simulink model "abl_M4_rigidPPC"  (R2023b)
settings: Solver=ode45  StartTime=0.0  StopTime=80  MaxStep=1e-3  RelTol=5e-5
model workspace (MAT data in the model file):
  gpsid1 = Simulink.Signal
  gpsid1.DataType = 'double'
  gpsid1.Dimensions = 1
  gpsid1.DimensionsMode = 'auto'
  gpsid1.Complexity = 'real'
  gpsid1.SampleTime = -1
  gpsid1.SamplingMode = 'auto'
  gpsid2 = Simulink.Signal
  gpsid2.DataType = 'double'
  gpsid2.Dimensions = 1
  gpsid2.DimensionsMode = 'auto'
  gpsid2.Complexity = 'real'
  gpsid2.SampleTime = -1
  gpsid2.SamplingMode = 'auto'
  gpsid3 = Simulink.Signal
  gpsid3.DataType = 'double'
  gpsid3.Dimensions = 1
  gpsid3.DimensionsMode = 'auto'
  gpsid3.Complexity = 'real'
  gpsid3.SampleTime = -1
  gpsid3.SamplingMode = 'auto'
  kkk1 = Simulink.Signal
  kkk1.DataType = 'double'
  kkk1.Dimensions = 1
  kkk1.DimensionsMode = 'auto'
  kkk1.Complexity = 'real'
  kkk1.SampleTime = -1
  kkk1.SamplingMode = 'auto'
  kkk2 = Simulink.Signal
  kkk2.DataType = 'double'
  kkk2.Dimensions = 1
  kkk2.DimensionsMode = 'auto'
  kkk2.Complexity = 'real'
  kkk2.SampleTime = -1
  kkk2.SamplingMode = 'auto'
  kkk3 = Simulink.Signal
  kkk3.DataType = 'double'
  kkk3.Dimensions = 1
  kkk3.DimensionsMode = 'auto'
  kkk3.Complexity = 'real'
  kkk3.SampleTime = -1
  kkk3.SamplingMode = 'auto'
  psid = 0.5
undefined symbols (not defined in the file): A_raw1, A_raw2, beta1, beta2, p00, p_d_10, p_d_20, p_d_30, p_d_40, p_d_50, p_d_60, p_hat_p10, p_hat_p20, p_hat_p30, p_hat_p40, p_hat_p50, p_hat_p60, p_hat_v10, p_hat_v20, p_hat_v30, p_hat_v40, p_hat_v50, p_hat_v60, p_off_set1, p_off_set2, v00
(part 1 of 4)
settings Model: Creator=ROG  LastModifiedBy=Administrator
settings SolverCC: MaxConsecutiveMinStep=5

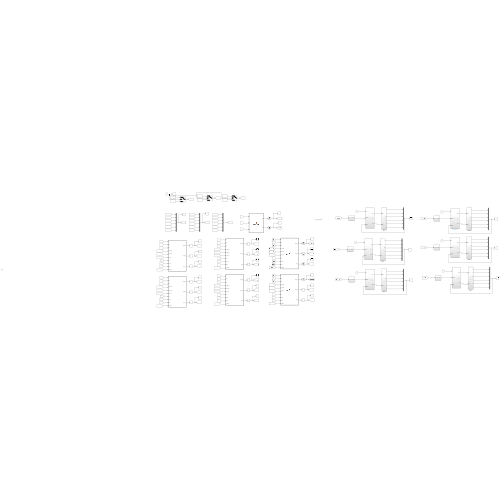
[thumbnail: Simulink's stored preview of the top-level diagram]
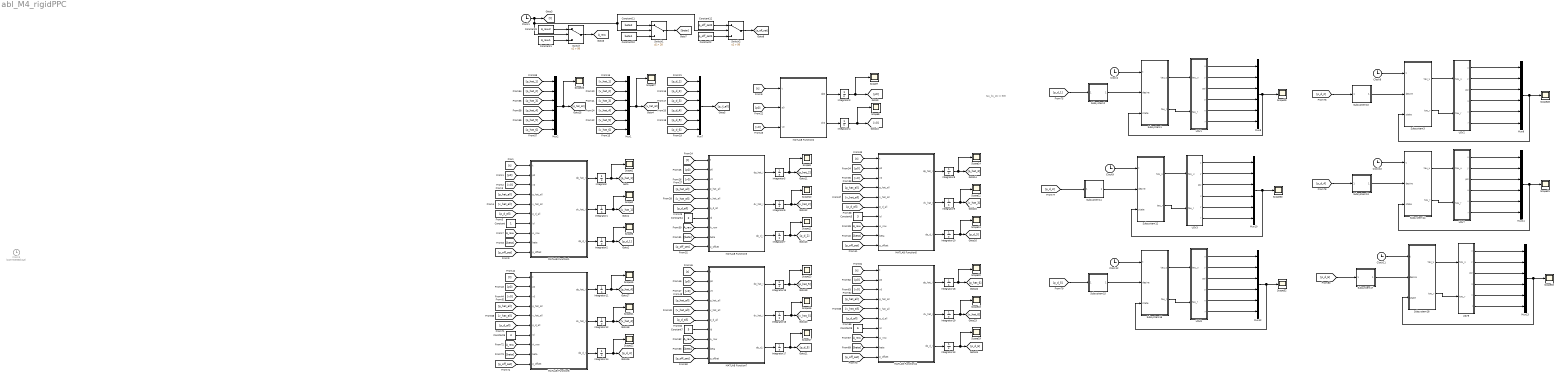
== system abl_M4_rigidPPC ==
  note: tau_bu_psi = 500
  note: l
  Clock{1..2,8..12} (7 alike) : Clock
  Clock3 : Clock  Commented=on
  Constant : Constant
  Constant1 : Constant  Value=A_raw1
  Constant10 : Constant  Value=beta1
  Constant11 : Constant  Value=beta2
  Constant12 : Constant  Value=p_off_set2
  Constant2 : Constant  Value=p_off_set1
  Constant4 : Constant  Value=2
  Constant5 : Constant  Value=3
  Constant6 : Constant  Value=4
  Constant7 : Constant  Value=5
  Constant8 : Constant  Value=6
  Constant9 : Constant  Value=A_raw2
  Integrator : Integrator  InitialCondition=p_hat_p10
  Integrator1 : Integrator  InitialCondition=p_hat_v10
  Integrator10 : Integrator  InitialCondition=p_d_30
  Integrator11 : Integrator  InitialCondition=p_hat_p40
  Integrator12 : Integrator  InitialCondition=p_hat_v40
  Integrator13 : Integrator  InitialCondition=p_d_60
  Integrator14 : Integrator  InitialCondition=p_d_40
  Integrator15 : Integrator  InitialCondition=p_hat_p50
  Integrator16 : Integrator  InitialCondition=p_hat_v50
  Integrator17 : Integrator  InitialCondition=p_d_50
  Integrator18 : Integrator  InitialCondition=p_hat_p60
  Integrator19 : Integrator  InitialCondition=p_hat_v60
  Integrator2 : Integrator  InitialCondition=p_d_10
  Integrator3 : Integrator  InitialCondition=p00
  Integrator4 : Integrator  InitialCondition=v00
  Integrator5 : Integrator  InitialCondition=p_hat_p20
  Integrator6 : Integrator  InitialCondition=p_hat_v20
  Integrator7 : Integrator  InitialCondition=p_d_20
  Integrator8 : Integrator  InitialCondition=p_hat_p30
  Integrator9 : Integrator  InitialCondition=p_hat_v30
  MATLAB Function1 : MATLAB Function  TreatAsAtomicUnit=on
  MATLAB Function11 : MATLAB Function  TreatAsAtomicUnit=on
  MATLAB Function2 : MATLAB Function  TreatAsAtomicUnit=on
  MATLAB Function3 : MATLAB Function  TreatAsAtomicUnit=on
  MATLAB Function5 : MATLAB Function  TreatAsAtomicUnit=on
  MATLAB Function6 : MATLAB Function  TreatAsAtomicUnit=on
  MATLAB Function7 : MATLAB Function  TreatAsAtomicUnit=on
  Mux{1..2,7..13} (9 alike) : Mux  Inputs=6
  Scope{1..2,6..23,26..33} (28 alike) : Scope
  Subsystem1 : Subsystem
  Subsystem10 : Subsystem
  Subsystem11 : Subsystem
  Subsystem12 : Subsystem
  Subsystem13 : Subsystem
  Subsystem14 : Subsystem
  Subsystem15 : Subsystem
  Subsystem16 : Subsystem
  Subsystem17 : Subsystem
  Subsystem18 : Subsystem
  Subsystem2 : Subsystem
  Subsystem3 : Subsystem
  Switch : Switch  Criteria=u2 > Threshold  Threshold=50  SaturateOnIntegerOverflow=off  InputSameDT=off
  Switch1 : Switch  Criteria=u2 > Threshold  Threshold=20  SaturateOnIntegerOverflow=off  InputSameDT=off
  Switch2 : Switch  Criteria=u2 > Threshold  Threshold=50  SaturateOnIntegerOverflow=off  InputSameDT=off
  USV1 : Subsystem
  USV2 : Subsystem
  USV3 : Subsystem
  USV7 : Subsystem
  USV8 : Subsystem
  USV9 : Subsystem
  tag scope: A_raw=global
  wires:
  MATLAB Function1/1(dp_hat_i) -> Integrator/1
  MATLAB Function1/2(dv_hat_i) -> Integrator1/1
  MATLAB Function1/3(dp_d_i) -> Integrator2/1
  Integrator/1 -> Scope1/1, [p_hat_1]
  Integrator1/1 -> Scope2/1, [v_hat_1]
  Integrator2/1 -> Scope6/1, [p_d_1]
  [t] -> MATLAB Function1/1(t)
  [p0] -> MATLAB Function1/2(p0)
  [v0] -> MATLAB Function1/3(v0)
  [p_hat_all] -> MATLAB Function1/4(p_hat_all)
  [v_hat_all] -> MATLAB Function1/5(v_hat_all)
  [p_d_all] -> MATLAB Function1/6(p_d_all)
  Constant/1 -> MATLAB Function1/7(id)
  [A_raw] -> MATLAB Function1/8(A_row)
  [beta] -> MATLAB Function1/9(beta)
  [p_off_set] -> MATLAB Function1/10(p_offset)
  [p_hat_3] -> Mux2/3
  [p_hat_1] -> Mux2/1
  [p_hat_6] -> Mux2/6
  [p_hat_4] -> Mux2/4
  [p_hat_5] -> Mux2/5
  Mux2/1 -> Scope26/1, [p_hat_all]
  [p_hat_2] -> Mux2/2
  [v_hat_1] -> Mux1/1
  [v_hat_4] -> Mux1/4
  [v_hat_2] -> Mux1/2
  [v_hat_6] -> Mux1/6
  Mux1/1 -> Scope27/1, [v_hat_all]
  [v_hat_5] -> Mux1/5
  [v_hat_3] -> Mux1/3
  [p_d_5] -> Mux7/5
  [p_d_4] -> Mux7/4
  [p_d_6] -> Mux7/6
  [p_d_2] -> Mux7/2
  Mux7/1 -> [p_d_all]
  [p_d_1] -> Mux7/1
  [p_d_3] -> Mux7/3
  MATLAB Function2/1(dp0) -> Integrator3/1
  MATLAB Function2/2(dv0) -> Integrator4/1
  Integrator4/1 -> Scope8/1, [v0]
  Integrator3/1 -> Scope7/1, [p0]
  [t] -> MATLAB Function2/1(t)
  [p0] -> MATLAB Function2/2(p0)
  [v0] -> MATLAB Function2/3(v0)
  Integrator7/1 -> Scope11/1, [p_d_2]
  Integrator5/1 -> Scope9/1, [p_hat_2]
  Integrator6/1 -> Scope10/1, [v_hat_2]
  MATLAB Function3/2(dv_hat_i) -> Integrator6/1
  [p0] -> MATLAB Function3/2(p0)
  MATLAB Function3/1(dp_hat_i) -> Integrator5/1
  [t] -> MATLAB Function3/1(t)
  [p_off_set] -> MATLAB Function3/10(p_offset)
  [p_d_all] -> MATLAB Function3/6(p_d_all)
  [v_hat_all] -> MATLAB Function3/5(v_hat_all)
  [p_hat_all] -> MATLAB Function3/4(p_hat_all)
  Constant4/1 -> MATLAB Function3/7(id)
  [A_raw] -> MATLAB Function3/8(A_row)
  MATLAB Function3/3(dp_d_i) -> Integrator7/1
  [beta] -> MATLAB Function3/9(beta)
  [v0] -> MATLAB Function3/3(v0)
  [beta] -> MATLAB Function5/9(beta)
  Constant5/1 -> MATLAB Function5/7(id)
  [p_hat_all] -> MATLAB Function5/4(p_hat_all)
  MATLAB Function5/3(dp_d_i) -> Integrator10/1
  [A_raw] -> MATLAB Function5/8(A_row)
  [p_d_all] -> MATLAB Function5/6(p_d_all)
  [v_hat_all] -> MATLAB Function5/5(v_hat_all)
  Integrator9/1 -> Scope12/1, [v_hat_3]
  [p_off_set] -> MATLAB Function5/10(p_offset)
  MATLAB Function5/1(dp_hat_i) -> Integrator8/1
  MATLAB Function5/2(dv_hat_i) -> Integrator9/1
  Integrator8/1 -> Scope14/1, [p_hat_3]
  [p0] -> MATLAB Function5/2(p0)
  Integrator10/1 -> Scope13/1, [p_d_3]
  [v0] -> MATLAB Function5/3(v0)
  [t] -> MATLAB Function5/1(t)
  Integrator14/1 -> Scope22/1, [p_d_4]
  Integrator11/1 -> Scope15/1, [p_hat_4]
  Integrator12/1 -> Scope21/1, [v_hat_4]
  MATLAB Function6/2(dv_hat_i) -> Integrator12/1
  MATLAB Function6/1(dp_hat_i) -> Integrator11/1
  Integrator13/1 -> Scope19/1, [p_d_6]
  Integrator19/1 -> Scope18/1, [v_hat_6]
  [v_hat_all] -> MATLAB Function11/5(v_hat_all)
  [p_d_all] -> MATLAB Function11/6(p_d_all)
  [p0] -> MATLAB Function6/2(p0)
  [A_raw] -> MATLAB Function11/8(A_row)
  [p_hat_all] -> MATLAB Function11/4(p_hat_all)
  MATLAB Function11/3(dp_d_i) -> Integrator13/1
  Constant8/1 -> MATLAB Function11/7(id)
  [beta] -> MATLAB Function7/9(beta)
  Constant7/1 -> MATLAB Function7/7(id)
  [p_hat_all] -> MATLAB Function7/4(p_hat_all)
  MATLAB Function7/3(dp_d_i) -> Integrator17/1
  [p_d_all] -> MATLAB Function7/6(p_d_all)
  [v_hat_all] -> MATLAB Function7/5(v_hat_all)
  [t] -> MATLAB Function11/1(t)
  Integrator16/1 -> Scope16/1, [v_hat_5]
  [v0] -> MATLAB Function11/3(v0)
  MATLAB Function7/1(dp_hat_i) -> Integrator15/1
  [p_off_set] -> MATLAB Function11/10(p_offset)
  [p0] -> MATLAB Function11/2(p0)
  [t] -> MATLAB Function7/1(t)
  [p0] -> MATLAB Function7/2(p0)
  Integrator15/1 -> Scope23/1, [p_hat_5]
  MATLAB Function11/2(dv_hat_i) -> Integrator19/1
  Integrator18/1 -> Scope20/1, [p_hat_6]
  Integrator17/1 -> Scope17/1, [p_d_5]
  MATLAB Function11/1(dp_hat_i) -> Integrator18/1
  [v0] -> MATLAB Function7/3(v0)
  [p_off_set] -> MATLAB Function7/10(p_offset)
  [A_raw] -> MATLAB Function7/8(A_row)
  [t] -> MATLAB Function6/1(t)
  [p_d_all] -> MATLAB Function6/6(p_d_all)
  [p_off_set] -> MATLAB Function6/10(p_offset)
  [v_hat_all] -> MATLAB Function6/5(v_hat_all)
  [p_hat_all] -> MATLAB Function6/4(p_hat_all)
  Constant6/1 -> MATLAB Function6/7(id)
  [A_raw] -> MATLAB Function6/8(A_row)
  MATLAB Function6/3(dp_d_i) -> Integrator14/1
  [beta] -> MATLAB Function6/9(beta)
  MATLAB Function7/2(dv_hat_i) -> Integrator16/1
  [v0] -> MATLAB Function6/3(v0)
  [beta] -> MATLAB Function11/9(beta)
  Switch/1 -> [A_raw]
  Constant1/1 -> Switch/3
  Constant9/1 -> Switch/1
  Constant11/1 -> Switch1/1
  Switch1/1 -> [beta]
  Constant10/1 -> Switch1/3
  Constant2/1 -> Switch2/3
  Clock1/1 -> Switch2/2, Switch1/2, Switch/2, [t]
  Constant12/1 -> Switch2/1
  Switch2/1 -> [p_off_set]
  USV1/2(y) -> Mux8/2
  [p_d_1] -> Subsystem2/1(p1_hat)
  USV1/4(u) -> Mux8/4
  USV1/1(x) -> Mux8/1
  Subsystem1/2(tau_r) -> USV1/2(tau_r)
  USV1/6(r) -> Mux8/6
  Mux8/1 -> Scope29/1, Subsystem1/3(state)
  USV1/5(v) -> Mux8/5
  Clock2/1 -> Subsystem1/1(t)
  Subsystem1/1(tau_u) -> USV1/1(tau_u)
  USV1/3(psi) -> Mux8/3
  Subsystem2/1(desire) -> Subsystem1/2(desire)
  USV2/1(x) -> Mux9/1
  Subsystem10/1(desire) -> Subsystem3/2(desire)
  Mux9/1 -> Scope28/1, Subsystem3/3(state)
  USV2/3(psi) -> Mux9/3
  Subsystem3/2(tau_r) -> USV2/2(tau_r)
  [p_d_2] -> Subsystem10/1(p1_hat)
  Clock8/1 -> Subsystem3/1(t)
  USV2/5(v) -> Mux9/5
  Subsystem3/1(tau_u) -> USV2/1(tau_u)
  USV2/6(r) -> Mux9/6
  USV2/4(u) -> Mux9/4
  USV2/2(y) -> Mux9/2
  Mux10/1 -> Scope30/1, Subsystem12/3(state)
  Clock9/1 -> Subsystem12/1(t)
  USV3/3(psi) -> Mux10/3
  Subsystem12/2(tau_r) -> USV3/2(tau_r)
  USV3/4(u) -> Mux10/4
  USV3/2(y) -> Mux10/2
  Subsystem12/1(tau_u) -> USV3/1(tau_u)
  USV3/5(v) -> Mux10/5
  USV3/6(r) -> Mux10/6
  Subsystem11/1(desire) -> Subsystem12/2(desire)
  USV3/1(x) -> Mux10/1
  USV7/2(y) -> Mux11/2
  Subsystem14/1(tau_u) -> USV7/1(tau_u)
  USV7/4(u) -> Mux11/4
  [p_d_4] -> Subsystem13/1(p1_hat)
  USV7/3(psi) -> Mux11/3
  Subsystem14/2(tau_r) -> USV7/2(tau_r)
  Mux11/1 -> Scope31/1, Subsystem14/3(state)
  Subsystem13/1(desire) -> Subsystem14/2(desire)
  USV7/1(x) -> Mux11/1
  USV7/6(r) -> Mux11/6
  Clock10/1 -> Subsystem14/1(t)
  USV7/5(v) -> Mux11/5
  Subsystem18/2(tau_r) -> USV9/2(tau_r)
  USV9/2(y) -> Mux13/2
  USV8/2(y) -> Mux12/2
  Subsystem16/1(tau_u) -> USV8/1(tau_u)
  USV8/4(u) -> Mux12/4
  Subsystem18/1(tau_u) -> USV9/1(tau_u)
  [p_d_5] -> Subsystem15/1(p1_hat)
  [p_d_6] -> Subsystem17/1(p1_hat)
  USV8/3(psi) -> Mux12/3
  Subsystem16/2(tau_r) -> USV8/2(tau_r)
  Clock12/1 -> Subsystem16/1(t)
  Mux12/1 -> Scope32/1, Subsystem16/3(state)
  USV9/3(psi) -> Mux13/3
  Subsystem17/1(desire) -> Subsystem18/2(desire)
  USV9/1(x) -> Mux13/1
  Subsystem15/1(desire) -> Subsystem16/2(desire)
  Mux13/1 -> Scope33/1, Subsystem18/3(state)
  USV8/1(x) -> Mux12/1
  USV9/6(r) -> Mux13/6
  USV8/6(r) -> Mux12/6
  USV9/5(v) -> Mux13/5
  USV9/4(u) -> Mux13/4
  Clock11/1 -> Subsystem18/1(t)
  USV8/5(v) -> Mux12/5
  [p_d_3] -> Subsystem11/1(p1_hat)

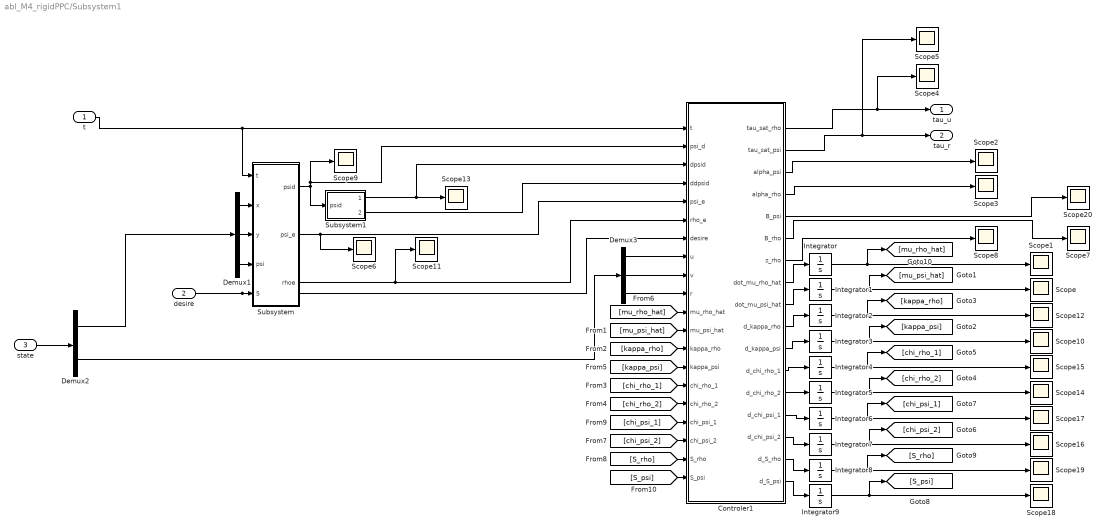
== system abl_M4_rigidPPC/Subsystem1 ==
  t : Inport
  desire : Inport  Port=2
  state : Inport  Port=3
  Controler1 : MATLAB Function  TreatAsAtomicUnit=on
  Demux1 : Demux  Outputs=3
  Demux2 : Demux  Outputs=2
  Demux3 : Demux  Outputs=3
  Integrator{,1..9} (10 alike) : Integrator  InitialCondition=0.1
  Scope{,1..20} (21 alike) : Scope
  Subsystem : Subsystem
  Subsystem1 : Subsystem
  tau_u : Outport
  tau_r : Outport  Port=2
  wires:
  desire/1 -> Controler1/7(desire), Subsystem/5("desire ")
  Demux1/1 -> Subsystem/2(x)
  Subsystem/1(psid) -> Scope9/1, Controler1/2(psi_d), Subsystem1/1(psid)
  Subsystem1/2(ddpsid) -> Controler1/4(ddpsid)
  Subsystem/3(rhoe) -> Scope11/1, Controler1/6(rho_e)
  Demux1/3 -> Subsystem/4(psi)
  t/1 -> Subsystem/1(t), Controler1/1(t)
  Demux1/2 -> Subsystem/3(y)
  Demux2/1 -> Demux1/1
  Subsystem1/1(dpsid) -> Scope13/1, Controler1/3(dpsid)
  Subsystem/2(psi_e) -> Scope6/1, Controler1/5(psi_e)
  state/1 -> Demux2/1
  Integrator/1 -> [mu_rho_hat], Scope1/1
  Controler1/4(alpha_rho) -> Scope3/1
  Controler1/2(tau_sat_psi) -> tau_r/1, Scope5/1
  Controler1/8(dot_mu_rho_hat) -> Integrator/1
  Controler1/1(tau_sat_rho) -> tau_u/1, Scope4/1
  Controler1/3(alpha_psi) -> Scope2/1
  Controler1/9(dot_mu_psi_hat) -> Integrator1/1
  Integrator1/1 -> [mu_psi_hat], Scope/1
  Controler1/6(B_rho) -> Scope7/1
  Controler1/7(z_rho) -> Scope8/1
  Demux2/2 -> Demux3/1
  Demux3/2 -> Controler1/9(v)
  Demux3/1 -> Controler1/8(u)
  Demux3/3 -> Controler1/10(r)
  Controler1/11(d_kappa_psi) -> Integrator3/1
  Controler1/10(d_kappa_rho) -> Integrator2/1
  Integrator3/1 -> [kappa_psi], Scope10/1
  Integrator2/1 -> [kappa_rho], Scope12/1
  Controler1/13(d_chi_rho_2) -> Integrator5/1
  Controler1/12(d_chi_rho_1) -> Integrator4/1
  Integrator5/1 -> [chi_rho_2], Scope14/1
  Integrator4/1 -> [chi_rho_1], Scope15/1
  Controler1/15(d_chi_psi_2) -> Integrator7/1
  Controler1/14(d_chi_psi_1) -> Integrator6/1
  Integrator7/1 -> [chi_psi_2], Scope16/1
  Integrator6/1 -> [chi_psi_1], Scope17/1
  Controler1/17(d_S_psi) -> Integrator9/1
  Controler1/16(d_S_rho) -> Integrator8/1
  Integrator9/1 -> [S_psi], Scope18/1
  Integrator8/1 -> [S_rho], Scope19/1
  [mu_rho_hat] -> Controler1/11(mu_rho_hat)
  [mu_psi_hat] -> Controler1/12(mu_psi_hat)
  [kappa_rho] -> Controler1/13(kappa_rho)
  [chi_rho_2] -> Controler1/16(chi_rho_2)
  [chi_rho_1] -> Controler1/15(chi_rho_1)
  [kappa_psi] -> Controler1/14(kappa_psi)
  [S_rho] -> Controler1/19(S_rho)
  [chi_psi_2] -> Controler1/18(chi_psi_2)
  [chi_psi_1] -> Controler1/17(chi_psi_1)
  [S_psi] -> Controler1/20(S_psi)
  Controler1/5(B_psi) -> Scope20/1

== system abl_M4_rigidPPC/Subsystem10 ==
  p1_hat : Inport
  Demux : Demux  Outputs=2
  Demux1 : Demux  Outputs=2
  Demux2 : Demux  Outputs=2
  Integrator{,1..3} (4 alike) : Integrator
  MATLAB Function8 : MATLAB Function  TreatAsAtomicUnit=on
  MATLAB Function9 : MATLAB Function  TreatAsAtomicUnit=on
  Mux7 : Mux  Inputs=6
  Scope : Scope
  desire : Outport
  wires:
  Demux/2 -> Mux7/4
  MATLAB Function9/2(dotx2) -> Integrator1/1
  MATLAB Function9/1(dotx1) -> Integrator/1
  Demux/1 -> Mux7/1
  Demux2/1 -> Mux7/3
  MATLAB Function8/2(dotx2) -> Integrator3/1
  Demux2/2 -> Mux7/6
  p1_hat/1 -> MATLAB Function9/3(pd), Scope/1, Demux/1
  Demux1/1 -> Mux7/2
  Integrator3/1 -> Demux2/1, MATLAB Function8/2(x2)
  MATLAB Function8/1(dotx1) -> Integrator2/1
  Integrator/1 -> MATLAB Function9/1(x1)
  Mux7/1 -> desire/1
  Integrator1/1 -> MATLAB Function8/3(dpd), Demux1/1, MATLAB Function9/2(x2)
  Integrator2/1 -> MATLAB Function8/1(x1)
  Demux1/2 -> Mux7/5

== system abl_M4_rigidPPC/Subsystem11 ==
  p1_hat : Inport
  Demux : Demux  Outputs=2
  Demux1 : Demux  Outputs=2
  Demux2 : Demux  Outputs=2
  Integrator{,1..3} (4 alike) : Integrator
  MATLAB Function8 : MATLAB Function  TreatAsAtomicUnit=on
  MATLAB Function9 : MATLAB Function  TreatAsAtomicUnit=on
  Mux7 : Mux  Inputs=6
  Scope : Scope
  desire : Outport
  wires:
  Demux/2 -> Mux7/4
  MATLAB Function9/2(dotx2) -> Integrator1/1
  MATLAB Function9/1(dotx1) -> Integrator/1
  Demux/1 -> Mux7/1
  Demux2/1 -> Mux7/3
  MATLAB Function8/2(dotx2) -> Integrator3/1
  Demux2/2 -> Mux7/6
  p1_hat/1 -> MATLAB Function9/3(pd), Scope/1, Demux/1
  Demux1/1 -> Mux7/2
  Integrator3/1 -> Demux2/1, MATLAB Function8/2(x2)
  MATLAB Function8/1(dotx1) -> Integrator2/1
  Integrator/1 -> MATLAB Function9/1(x1)
  Mux7/1 -> desire/1
  Integrator1/1 -> MATLAB Function8/3(dpd), Demux1/1, MATLAB Function9/2(x2)
  Integrator2/1 -> MATLAB Function8/1(x1)
  Demux1/2 -> Mux7/5

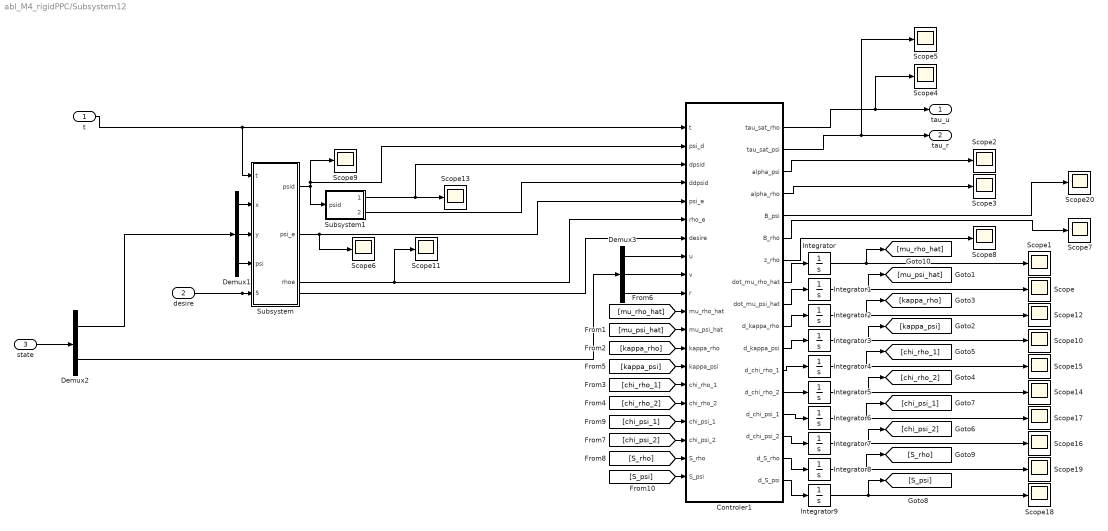
== system abl_M4_rigidPPC/Subsystem12 ==
  t : Inport
  desire : Inport  Port=2
  state : Inport  Port=3
  Controler1 : MATLAB Function  TreatAsAtomicUnit=on
  Demux1 : Demux  Outputs=3
  Demux2 : Demux  Outputs=2
  Demux3 : Demux  Outputs=3
  Integrator{,1..9} (10 alike) : Integrator  InitialCondition=0.1
  Scope{,1..20} (21 alike) : Scope
  Subsystem : Subsystem
  Subsystem1 : Subsystem
  tau_u : Outport
  tau_r : Outport  Port=2
  wires:
  desire/1 -> Controler1/7(desire), Subsystem/5("desire ")
  Demux1/1 -> Subsystem/2(x)
  Subsystem/1(psid) -> Scope9/1, Controler1/2(psi_d), Subsystem1/1(psid)
  Subsystem1/2(ddpsid) -> Controler1/4(ddpsid)
  Subsystem/3(rhoe) -> Scope11/1, Controler1/6(rho_e)
  Demux1/3 -> Subsystem/4(psi)
  t/1 -> Subsystem/1(t), Controler1/1(t)
  Demux1/2 -> Subsystem/3(y)
  Demux2/1 -> Demux1/1
  Subsystem1/1(dpsid) -> Scope13/1, Controler1/3(dpsid)
  Subsystem/2(psi_e) -> Scope6/1, Controler1/5(psi_e)
  state/1 -> Demux2/1
  Integrator/1 -> [mu_rho_hat], Scope1/1
  Controler1/4(alpha_rho) -> Scope3/1
  Controler1/2(tau_sat_psi) -> tau_r/1, Scope5/1
  Controler1/8(dot_mu_rho_hat) -> Integrator/1
  Controler1/1(tau_sat_rho) -> tau_u/1, Scope4/1
  Controler1/3(alpha_psi) -> Scope2/1
  Controler1/9(dot_mu_psi_hat) -> Integrator1/1
  Integrator1/1 -> [mu_psi_hat], Scope/1
  Controler1/6(B_rho) -> Scope7/1
  Controler1/7(z_rho) -> Scope8/1
  Demux2/2 -> Demux3/1
  Demux3/2 -> Controler1/9(v)
  Demux3/1 -> Controler1/8(u)
  Demux3/3 -> Controler1/10(r)
  Controler1/11(d_kappa_psi) -> Integrator3/1
  Controler1/10(d_kappa_rho) -> Integrator2/1
  Integrator3/1 -> [kappa_psi], Scope10/1
  Integrator2/1 -> [kappa_rho], Scope12/1
  Controler1/13(d_chi_rho_2) -> Integrator5/1
  Controler1/12(d_chi_rho_1) -> Integrator4/1
  Integrator5/1 -> [chi_rho_2], Scope14/1
  Integrator4/1 -> [chi_rho_1], Scope15/1
  Controler1/15(d_chi_psi_2) -> Integrator7/1
  Controler1/14(d_chi_psi_1) -> Integrator6/1
  Integrator7/1 -> [chi_psi_2], Scope16/1
  Integrator6/1 -> [chi_psi_1], Scope17/1
  Controler1/17(d_S_psi) -> Integrator9/1
  Controler1/16(d_S_rho) -> Integrator8/1
  Integrator9/1 -> [S_psi], Scope18/1
  Integrator8/1 -> [S_rho], Scope19/1
  [mu_rho_hat] -> Controler1/11(mu_rho_hat)
  [mu_psi_hat] -> Controler1/12(mu_psi_hat)
  [kappa_rho] -> Controler1/13(kappa_rho)
  [chi_rho_2] -> Controler1/16(chi_rho_2)
  [chi_rho_1] -> Controler1/15(chi_rho_1)
  [kappa_psi] -> Controler1/14(kappa_psi)
  [S_rho] -> Controler1/19(S_rho)
  [chi_psi_2] -> Controler1/18(chi_psi_2)
  [chi_psi_1] -> Controler1/17(chi_psi_1)
  [S_psi] -> Controler1/20(S_psi)
  Controler1/5(B_psi) -> Scope20/1

== system abl_M4_rigidPPC/Subsystem13 ==
  p1_hat : Inport
  Demux : Demux  Outputs=2
  Demux1 : Demux  Outputs=2
  Demux2 : Demux  Outputs=2
  Integrator : Integrator  InitialCondition=p_d_40
  Integrator1 : Integrator
  Integrator2 : Integrator
  Integrator3 : Integrator
  MATLAB Function8 : MATLAB Function  TreatAsAtomicUnit=on
  MATLAB Function9 : MATLAB Function  TreatAsAtomicUnit=on
  Mux7 : Mux  Inputs=6
  Scope : Scope  NumInputPorts=2
  Scope1 : Scope
  desire : Outport
  wires:
  Demux/2 -> Mux7/4
  MATLAB Function9/2(dotx2) -> Integrator1/1
  MATLAB Function9/1(dotx1) -> Integrator/1
  Demux/1 -> Mux7/1
  Demux2/1 -> Mux7/3
  MATLAB Function8/2(dotx2) -> Integrator3/1
  Demux2/2 -> Mux7/6
  p1_hat/1 -> MATLAB Function9/3(pd), Scope/1
  Demux1/1 -> Mux7/2
  Integrator3/1 -> Demux2/1, MATLAB Function8/2(x2)
  MATLAB Function8/1(dotx1) -> Integrator2/1
  Integrator/1 -> Scope1/1, Demux/1, Scope/2, MATLAB Function9/1(x1)
  Mux7/1 -> desire/1
  Integrator1/1 -> MATLAB Function8/3(dpd), Demux1/1, MATLAB Function9/2(x2)
  Integrator2/1 -> MATLAB Function8/1(x1)
  Demux1/2 -> Mux7/5

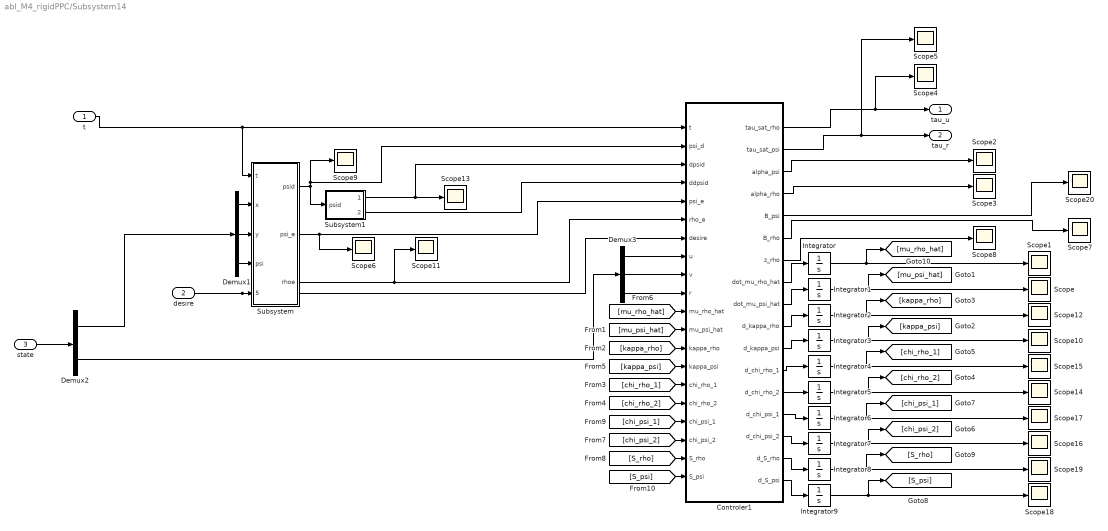
== system abl_M4_rigidPPC/Subsystem14 ==
  t : Inport
  desire : Inport  Port=2
  state : Inport  Port=3
  Controler1 : MATLAB Function  TreatAsAtomicUnit=on
  Demux1 : Demux  Outputs=3
  Demux2 : Demux  Outputs=2
  Demux3 : Demux  Outputs=3
  Integrator{,1..9} (10 alike) : Integrator  InitialCondition=0.1
  Scope{,1..20} (21 alike) : Scope
  Subsystem : Subsystem
  Subsystem1 : Subsystem
  tau_u : Outport
  tau_r : Outport  Port=2
  wires:
  desire/1 -> Controler1/7(desire), Subsystem/5("desire ")
  Demux1/1 -> Subsystem/2(x)
  Subsystem/1(psid) -> Scope9/1, Controler1/2(psi_d), Subsystem1/1(psid)
  Subsystem1/2(ddpsid) -> Controler1/4(ddpsid)
  Subsystem/3(rhoe) -> Scope11/1, Controler1/6(rho_e)
  Demux1/3 -> Subsystem/4(psi)
  t/1 -> Subsystem/1(t), Controler1/1(t)
  Demux1/2 -> Subsystem/3(y)
  Demux2/1 -> Demux1/1
  Subsystem1/1(dpsid) -> Scope13/1, Controler1/3(dpsid)
  Subsystem/2(psi_e) -> Scope6/1, Controler1/5(psi_e)
  state/1 -> Demux2/1
  Integrator/1 -> [mu_rho_hat], Scope1/1
  Controler1/4(alpha_rho) -> Scope3/1
  Controler1/2(tau_sat_psi) -> tau_r/1, Scope5/1
  Controler1/8(dot_mu_rho_hat) -> Integrator/1
  Controler1/1(tau_sat_rho) -> tau_u/1, Scope4/1
  Controler1/3(alpha_psi) -> Scope2/1
  Controler1/9(dot_mu_psi_hat) -> Integrator1/1
  Integrator1/1 -> [mu_psi_hat], Scope/1
  Controler1/6(B_rho) -> Scope7/1
  Controler1/7(z_rho) -> Scope8/1
  Demux2/2 -> Demux3/1
  Demux3/2 -> Controler1/9(v)
  Demux3/1 -> Controler1/8(u)
  Demux3/3 -> Controler1/10(r)
  Controler1/11(d_kappa_psi) -> Integrator3/1
  Controler1/10(d_kappa_rho) -> Integrator2/1
  Integrator3/1 -> [kappa_psi], Scope10/1
  Integrator2/1 -> [kappa_rho], Scope12/1
  Controler1/13(d_chi_rho_2) -> Integrator5/1
  Controler1/12(d_chi_rho_1) -> Integrator4/1
  Integrator5/1 -> [chi_rho_2], Scope14/1
  Integrator4/1 -> [chi_rho_1], Scope15/1
  Controler1/15(d_chi_psi_2) -> Integrator7/1
  Controler1/14(d_chi_psi_1) -> Integrator6/1
  Integrator7/1 -> [chi_psi_2], Scope16/1
  Integrator6/1 -> [chi_psi_1], Scope17/1
  Controler1/17(d_S_psi) -> Integrator9/1
  Controler1/16(d_S_rho) -> Integrator8/1
  Integrator9/1 -> [S_psi], Scope18/1
  Integrator8/1 -> [S_rho], Scope19/1
  [mu_rho_hat] -> Controler1/11(mu_rho_hat)
  [mu_psi_hat] -> Controler1/12(mu_psi_hat)
  [kappa_rho] -> Controler1/13(kappa_rho)
  [chi_rho_2] -> Controler1/16(chi_rho_2)
  [chi_rho_1] -> Controler1/15(chi_rho_1)
  [kappa_psi] -> Controler1/14(kappa_psi)
  [S_rho] -> Controler1/19(S_rho)
  [chi_psi_2] -> Controler1/18(chi_psi_2)
  [chi_psi_1] -> Controler1/17(chi_psi_1)
  [S_psi] -> Controler1/20(S_psi)
  Controler1/5(B_psi) -> Scope20/1

== system abl_M4_rigidPPC/Subsystem15 ==
  p1_hat : Inport
  Demux : Demux  Outputs=2
  Demux1 : Demux  Outputs=2
  Demux2 : Demux  Outputs=2
  Integrator{,1..3} (4 alike) : Integrator
  MATLAB Function8 : MATLAB Function  TreatAsAtomicUnit=on
  MATLAB Function9 : MATLAB Function  TreatAsAtomicUnit=on
  Mux7 : Mux  Inputs=6
  Scope : Scope
  desire : Outport
  wires:
  Demux/2 -> Mux7/4
  MATLAB Function9/2(dotx2) -> Integrator1/1
  MATLAB Function9/1(dotx1) -> Integrator/1
  Demux/1 -> Mux7/1
  Demux2/1 -> Mux7/3
  MATLAB Function8/2(dotx2) -> Integrator3/1
  Demux2/2 -> Mux7/6
  p1_hat/1 -> MATLAB Function9/3(pd), Scope/1, Demux/1
  Demux1/1 -> Mux7/2
  Integrator3/1 -> Demux2/1, MATLAB Function8/2(x2)
  MATLAB Function8/1(dotx1) -> Integrator2/1
  Integrator/1 -> MATLAB Function9/1(x1)
  Mux7/1 -> desire/1
  Integrator1/1 -> MATLAB Function8/3(dpd), Demux1/1, MATLAB Function9/2(x2)
  Integrator2/1 -> MATLAB Function8/1(x1)
  Demux1/2 -> Mux7/5

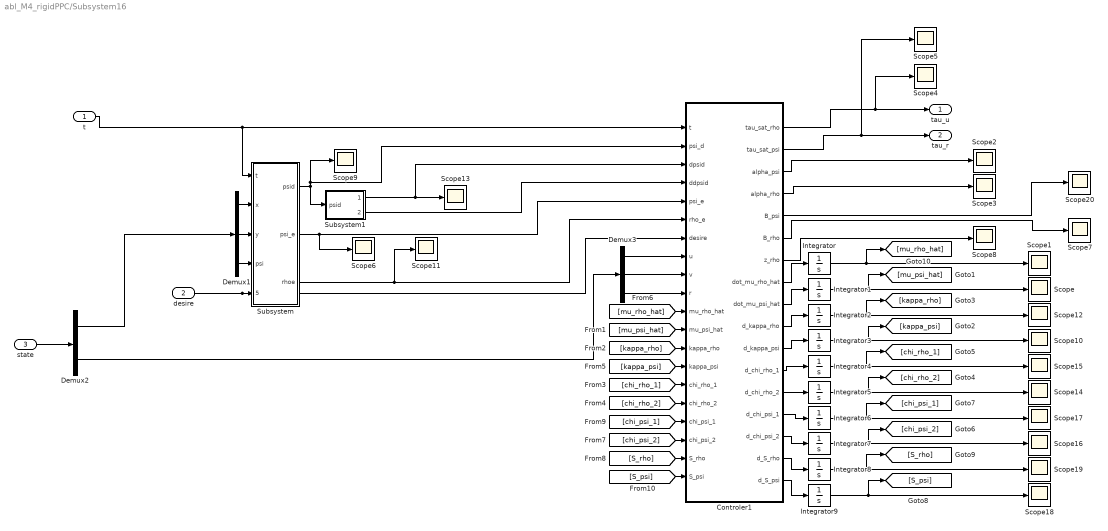
== system abl_M4_rigidPPC/Subsystem16 ==
  t : Inport
  desire : Inport  Port=2
  state : Inport  Port=3
  Controler1 : MATLAB Function  TreatAsAtomicUnit=on
  Demux1 : Demux  Outputs=3
  Demux2 : Demux  Outputs=2
  Demux3 : Demux  Outputs=3
  Integrator{,1..9} (10 alike) : Integrator  InitialCondition=0.1
  Scope{,1..20} (21 alike) : Scope
  Subsystem : Subsystem
  Subsystem1 : Subsystem
  tau_u : Outport
  tau_r : Outport  Port=2
  wires:
  desire/1 -> Controler1/7(desire), Subsystem/5("desire ")
  Demux1/1 -> Subsystem/2(x)
  Subsystem/1(psid) -> Scope9/1, Controler1/2(psi_d), Subsystem1/1(psid)
  Subsystem1/2(ddpsid) -> Controler1/4(ddpsid)
  Subsystem/3(rhoe) -> Scope11/1, Controler1/6(rho_e)
  Demux1/3 -> Subsystem/4(psi)
  t/1 -> Subsystem/1(t), Controler1/1(t)
  Demux1/2 -> Subsystem/3(y)
  Demux2/1 -> Demux1/1
  Subsystem1/1(dpsid) -> Scope13/1, Controler1/3(dpsid)
  Subsystem/2(psi_e) -> Scope6/1, Controler1/5(psi_e)
  state/1 -> Demux2/1
  Integrator/1 -> [mu_rho_hat], Scope1/1
  Controler1/4(alpha_rho) -> Scope3/1
  Controler1/2(tau_sat_psi) -> tau_r/1, Scope5/1
  Controler1/8(dot_mu_rho_hat) -> Integrator/1
  Controler1/1(tau_sat_rho) -> tau_u/1, Scope4/1
  Controler1/3(alpha_psi) -> Scope2/1
  Controler1/9(dot_mu_psi_hat) -> Integrator1/1
  Integrator1/1 -> [mu_psi_hat], Scope/1
  Controler1/6(B_rho) -> Scope7/1
  Controler1/7(z_rho) -> Scope8/1
  Demux2/2 -> Demux3/1
  Demux3/2 -> Controler1/9(v)
  Demux3/1 -> Controler1/8(u)
  Demux3/3 -> Controler1/10(r)
  Controler1/11(d_kappa_psi) -> Integrator3/1
  Controler1/10(d_kappa_rho) -> Integrator2/1
  Integrator3/1 -> [kappa_psi], Scope10/1
  Integrator2/1 -> [kappa_rho], Scope12/1
  Controler1/13(d_chi_rho_2) -> Integrator5/1
  Controler1/12(d_chi_rho_1) -> Integrator4/1
  Integrator5/1 -> [chi_rho_2], Scope14/1
  Integrator4/1 -> [chi_rho_1], Scope15/1
  Controler1/15(d_chi_psi_2) -> Integrator7/1
  Controler1/14(d_chi_psi_1) -> Integrator6/1
  Integrator7/1 -> [chi_psi_2], Scope16/1
  Integrator6/1 -> [chi_psi_1], Scope17/1
  Controler1/17(d_S_psi) -> Integrator9/1
  Controler1/16(d_S_rho) -> Integrator8/1
  Integrator9/1 -> [S_psi], Scope18/1
  Integrator8/1 -> [S_rho], Scope19/1
  [mu_rho_hat] -> Controler1/11(mu_rho_hat)
  [mu_psi_hat] -> Controler1/12(mu_psi_hat)
  [kappa_rho] -> Controler1/13(kappa_rho)
  [chi_rho_2] -> Controler1/16(chi_rho_2)
  [chi_rho_1] -> Controler1/15(chi_rho_1)
  [kappa_psi] -> Controler1/14(kappa_psi)
  [S_rho] -> Controler1/19(S_rho)
  [chi_psi_2] -> Controler1/18(chi_psi_2)
  [chi_psi_1] -> Controler1/17(chi_psi_1)
  [S_psi] -> Controler1/20(S_psi)
  Controler1/5(B_psi) -> Scope20/1

== system abl_M4_rigidPPC/Subsystem17 ==
  p1_hat : Inport
  Demux : Demux  Outputs=2
  Demux1 : Demux  Outputs=2
  Demux2 : Demux  Outputs=2
  Integrator{,1..3} (4 alike) : Integrator
  MATLAB Function8 : MATLAB Function  TreatAsAtomicUnit=on
  MATLAB Function9 : MATLAB Function  TreatAsAtomicUnit=on
  Mux7 : Mux  Inputs=6
  Scope : Scope
  desire : Outport
  wires:
  Demux/2 -> Mux7/4
  MATLAB Function9/2(dotx2) -> Integrator1/1
  MATLAB Function9/1(dotx1) -> Integrator/1
  Demux/1 -> Mux7/1
  Demux2/1 -> Mux7/3
  MATLAB Function8/2(dotx2) -> Integrator3/1
  Demux2/2 -> Mux7/6
  p1_hat/1 -> MATLAB Function9/3(pd), Scope/1, Demux/1
  Demux1/1 -> Mux7/2
  Integrator3/1 -> Demux2/1, MATLAB Function8/2(x2)
  MATLAB Function8/1(dotx1) -> Integrator2/1
  Integrator/1 -> MATLAB Function9/1(x1)
  Mux7/1 -> desire/1
  Integrator1/1 -> MATLAB Function8/3(dpd), Demux1/1, MATLAB Function9/2(x2)
  Integrator2/1 -> MATLAB Function8/1(x1)
  Demux1/2 -> Mux7/5

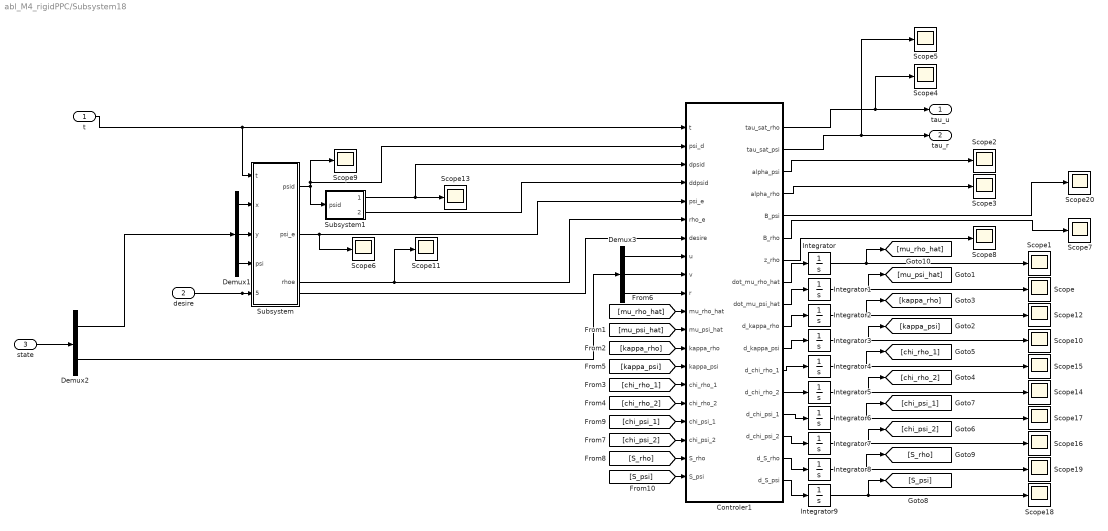
== system abl_M4_rigidPPC/Subsystem18 ==
  t : Inport
  desire : Inport  Port=2
  state : Inport  Port=3
  Controler1 : MATLAB Function  TreatAsAtomicUnit=on
  Demux1 : Demux  Outputs=3
  Demux2 : Demux  Outputs=2
  Demux3 : Demux  Outputs=3
  Integrator{,1..9} (10 alike) : Integrator  InitialCondition=0.1
  Scope{,1..20} (21 alike) : Scope
  Subsystem : Subsystem
  Subsystem1 : Subsystem
  tau_u : Outport
  tau_r : Outport  Port=2
  wires:
  desire/1 -> Controler1/7(desire), Subsystem/5("desire ")
  Demux1/1 -> Subsystem/2(x)
  Subsystem/1(psid) -> Scope9/1, Controler1/2(psi_d), Subsystem1/1(psid)
  Subsystem1/2(ddpsid) -> Controler1/4(ddpsid)
  Subsystem/3(rhoe) -> Scope11/1, Controler1/6(rho_e)
  Demux1/3 -> Subsystem/4(psi)
  t/1 -> Subsystem/1(t), Controler1/1(t)
  Demux1/2 -> Subsystem/3(y)
  Demux2/1 -> Demux1/1
  Subsystem1/1(dpsid) -> Scope13/1, Controler1/3(dpsid)
  Subsystem/2(psi_e) -> Scope6/1, Controler1/5(psi_e)
  state/1 -> Demux2/1
  Integrator/1 -> [mu_rho_hat], Scope1/1
  Controler1/4(alpha_rho) -> Scope3/1
  Controler1/2(tau_sat_psi) -> tau_r/1, Scope5/1
  Controler1/8(dot_mu_rho_hat) -> Integrator/1
  Controler1/1(tau_sat_rho) -> tau_u/1, Scope4/1
  Controler1/3(alpha_psi) -> Scope2/1
  Controler1/9(dot_mu_psi_hat) -> Integrator1/1
  Integrator1/1 -> [mu_psi_hat], Scope/1
  Controler1/6(B_rho) -> Scope7/1
  Controler1/7(z_rho) -> Scope8/1
  Demux2/2 -> Demux3/1
  Demux3/2 -> Controler1/9(v)
  Demux3/1 -> Controler1/8(u)
  Demux3/3 -> Controler1/10(r)
  Controler1/11(d_kappa_psi) -> Integrator3/1
  Controler1/10(d_kappa_rho) -> Integrator2/1
  Integrator3/1 -> [kappa_psi], Scope10/1
  Integrator2/1 -> [kappa_rho], Scope12/1
  Controler1/13(d_chi_rho_2) -> Integrator5/1
  Controler1/12(d_chi_rho_1) -> Integrator4/1
  Integrator5/1 -> [chi_rho_2], Scope14/1
  Integrator4/1 -> [chi_rho_1], Scope15/1
  Controler1/15(d_chi_psi_2) -> Integrator7/1
  Controler1/14(d_chi_psi_1) -> Integrator6/1
  Integrator7/1 -> [chi_psi_2], Scope16/1
  Integrator6/1 -> [chi_psi_1], Scope17/1
  Controler1/17(d_S_psi) -> Integrator9/1
  Controler1/16(d_S_rho) -> Integrator8/1
  Integrator9/1 -> [S_psi], Scope18/1
  Integrator8/1 -> [S_rho], Scope19/1
  [mu_rho_hat] -> Controler1/11(mu_rho_hat)
  [mu_psi_hat] -> Controler1/12(mu_psi_hat)
  [kappa_rho] -> Controler1/13(kappa_rho)
  [chi_rho_2] -> Controler1/16(chi_rho_2)
  [chi_rho_1] -> Controler1/15(chi_rho_1)
  [kappa_psi] -> Controler1/14(kappa_psi)
  [S_rho] -> Controler1/19(S_rho)
  [chi_psi_2] -> Controler1/18(chi_psi_2)
  [chi_psi_1] -> Controler1/17(chi_psi_1)
  [S_psi] -> Controler1/20(S_psi)
  Controler1/5(B_psi) -> Scope20/1

== system abl_M4_rigidPPC/Subsystem2 ==
  p1_hat : Inport
  Demux : Demux  Outputs=2
  Demux1 : Demux  Outputs=2
  Demux2 : Demux  Outputs=2
  Integrator{,1..3} (4 alike) : Integrator
  MATLAB Function8 : MATLAB Function  TreatAsAtomicUnit=on
  MATLAB Function9 : MATLAB Function  TreatAsAtomicUnit=on
  Mux7 : Mux  Inputs=6
  Scope : Scope
  desire : Outport
  wires:
  Demux/2 -> Mux7/4
  MATLAB Function9/2(dotx2) -> Integrator1/1
  MATLAB Function9/1(dotx1) -> Integrator/1
  Demux/1 -> Mux7/1
  Demux2/1 -> Mux7/3
  MATLAB Function8/2(dotx2) -> Integrator3/1
  Demux2/2 -> Mux7/6
  p1_hat/1 -> MATLAB Function9/3(pd), Scope/1, Demux/1
  Demux1/1 -> Mux7/2
  Integrator3/1 -> Demux2/1, MATLAB Function8/2(x2)
  MATLAB Function8/1(dotx1) -> Integrator2/1
  Integrator/1 -> MATLAB Function9/1(x1)
  Mux7/1 -> desire/1
  Integrator1/1 -> MATLAB Function8/3(dpd), Demux1/1, MATLAB Function9/2(x2)
  Integrator2/1 -> MATLAB Function8/1(x1)
  Demux1/2 -> Mux7/5

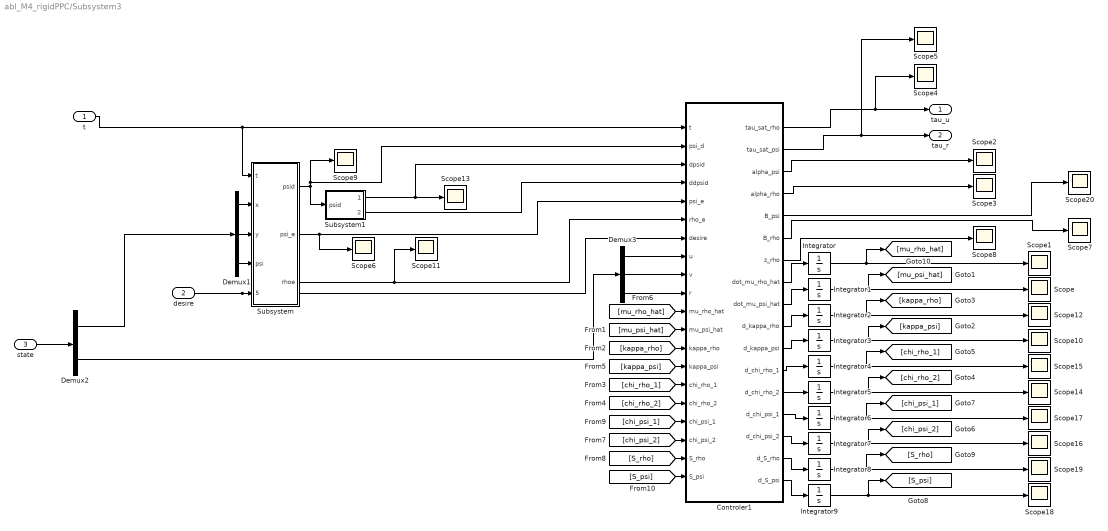
== system abl_M4_rigidPPC/Subsystem3 ==
  t : Inport
  desire : Inport  Port=2
  state : Inport  Port=3
  Controler1 : MATLAB Function  TreatAsAtomicUnit=on
  Demux1 : Demux  Outputs=3
  Demux2 : Demux  Outputs=2
  Demux3 : Demux  Outputs=3
  Integrator{,1..9} (10 alike) : Integrator  InitialCondition=0.1
  Scope{,1..20} (21 alike) : Scope
  Subsystem : Subsystem
  Subsystem1 : Subsystem
  tau_u : Outport
  tau_r : Outport  Port=2
  wires:
  desire/1 -> Controler1/7(desire), Subsystem/5("desire ")
  Demux1/1 -> Subsystem/2(x)
  Subsystem/1(psid) -> Scope9/1, Controler1/2(psi_d), Subsystem1/1(psid)
  Subsystem1/2(ddpsid) -> Controler1/4(ddpsid)
  Subsystem/3(rhoe) -> Scope11/1, Controler1/6(rho_e)
  Demux1/3 -> Subsystem/4(psi)
  t/1 -> Subsystem/1(t), Controler1/1(t)
  Demux1/2 -> Subsystem/3(y)
  Demux2/1 -> Demux1/1
  Subsystem1/1(dpsid) -> Scope13/1, Controler1/3(dpsid)
  Subsystem/2(psi_e) -> Scope6/1, Controler1/5(psi_e)
  state/1 -> Demux2/1
  Integrator/1 -> [mu_rho_hat], Scope1/1
  Controler1/4(alpha_rho) -> Scope3/1
  Controler1/2(tau_sat_psi) -> tau_r/1, Scope5/1
  Controler1/8(dot_mu_rho_hat) -> Integrator/1
  Controler1/1(tau_sat_rho) -> tau_u/1, Scope4/1
  Controler1/3(alpha_psi) -> Scope2/1
  Controler1/9(dot_mu_psi_hat) -> Integrator1/1
  Integrator1/1 -> [mu_psi_hat], Scope/1
  Controler1/6(B_rho) -> Scope7/1
  Controler1/7(z_rho) -> Scope8/1
  Demux2/2 -> Demux3/1
  Demux3/2 -> Controler1/9(v)
  Demux3/1 -> Controler1/8(u)
  Demux3/3 -> Controler1/10(r)
  Controler1/11(d_kappa_psi) -> Integrator3/1
  Controler1/10(d_kappa_rho) -> Integrator2/1
  Integrator3/1 -> [kappa_psi], Scope10/1
  Integrator2/1 -> [kappa_rho], Scope12/1
  Controler1/13(d_chi_rho_2) -> Integrator5/1
  Controler1/12(d_chi_rho_1) -> Integrator4/1
  Integrator5/1 -> [chi_rho_2], Scope14/1
  Integrator4/1 -> [chi_rho_1], Scope15/1
  Controler1/15(d_chi_psi_2) -> Integrator7/1
  Controler1/14(d_chi_psi_1) -> Integrator6/1
  Integrator7/1 -> [chi_psi_2], Scope16/1
  Integrator6/1 -> [chi_psi_1], Scope17/1
  Controler1/17(d_S_psi) -> Integrator9/1
  Controler1/16(d_S_rho) -> Integrator8/1
  Integrator9/1 -> [S_psi], Scope18/1
  Integrator8/1 -> [S_rho], Scope19/1
  [mu_rho_hat] -> Controler1/11(mu_rho_hat)
  [mu_psi_hat] -> Controler1/12(mu_psi_hat)
  [kappa_rho] -> Controler1/13(kappa_rho)
  [chi_rho_2] -> Controler1/16(chi_rho_2)
  [chi_rho_1] -> Controler1/15(chi_rho_1)
  [kappa_psi] -> Controler1/14(kappa_psi)
  [S_rho] -> Controler1/19(S_rho)
  [chi_psi_2] -> Controler1/18(chi_psi_2)
  [chi_psi_1] -> Controler1/17(chi_psi_1)
  [S_psi] -> Controler1/20(S_psi)
  Controler1/5(B_psi) -> Scope20/1

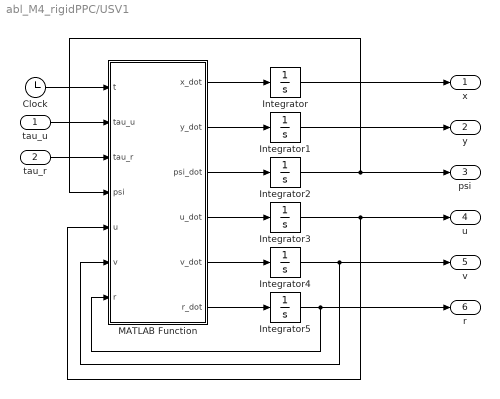
== system abl_M4_rigidPPC/USV1 ==
  tau_u : Inport
  tau_r : Inport  Port=2
  Clock : Clock
  Integrator : Integrator  InitialCondition=p_d_10(1)+8
  Integrator1 : Integrator  InitialCondition=p_d_10(2)+2
  Integrator{2..5} (4 alike) : Integrator
  MATLAB Function : MATLAB Function  TreatAsAtomicUnit=on
  x : Outport
  y : Outport  Port=2
  psi : Outport  Port=3
  u : Outport  Port=4
  v : Outport  Port=5
  r : Outport  Port=6
  wires:
  Integrator2/1 -> psi/1, MATLAB Function/4(psi)
  MATLAB Function/2(y_dot) -> Integrator1/1
  Integrator3/1 -> u/1, MATLAB Function/5(u)
  MATLAB Function/5(v_dot) -> Integrator4/1
  Integrator5/1 -> r/1, MATLAB Function/7(r)
  MATLAB Function/3(psi_dot) -> Integrator2/1
  MATLAB Function/6(r_dot) -> Integrator5/1
  tau_r/1 -> MATLAB Function/3(tau_r)
  Integrator4/1 -> v/1, MATLAB Function/6(v)
  Integrator/1 -> x/1
  MATLAB Function/4(u_dot) -> Integrator3/1
  MATLAB Function/1(x_dot) -> Integrator/1
  tau_u/1 -> MATLAB Function/2(tau_u)
  Integrator1/1 -> y/1
  Clock/1 -> MATLAB Function/1(t)

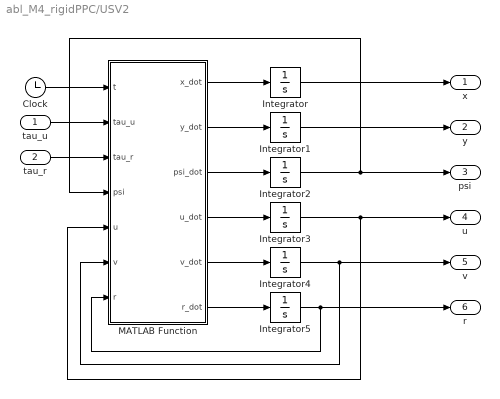
== system abl_M4_rigidPPC/USV2 ==
  tau_u : Inport
  tau_r : Inport  Port=2
  Clock : Clock
  Integrator : Integrator  InitialCondition=p_d_20(1)+8
  Integrator1 : Integrator  InitialCondition=p_d_20(2)+2
  Integrator{2..5} (4 alike) : Integrator
  MATLAB Function : MATLAB Function  TreatAsAtomicUnit=on
  x : Outport
  y : Outport  Port=2
  psi : Outport  Port=3
  u : Outport  Port=4
  v : Outport  Port=5
  r : Outport  Port=6
  wires:
  Integrator2/1 -> psi/1, MATLAB Function/4(psi)
  MATLAB Function/2(y_dot) -> Integrator1/1
  Integrator3/1 -> u/1, MATLAB Function/5(u)
  MATLAB Function/5(v_dot) -> Integrator4/1
  Integrator5/1 -> r/1, MATLAB Function/7(r)
  MATLAB Function/3(psi_dot) -> Integrator2/1
  MATLAB Function/6(r_dot) -> Integrator5/1
  tau_r/1 -> MATLAB Function/3(tau_r)
  Integrator4/1 -> v/1, MATLAB Function/6(v)
  Integrator/1 -> x/1
  MATLAB Function/4(u_dot) -> Integrator3/1
  MATLAB Function/1(x_dot) -> Integrator/1
  tau_u/1 -> MATLAB Function/2(tau_u)
  Integrator1/1 -> y/1
  Clock/1 -> MATLAB Function/1(t)

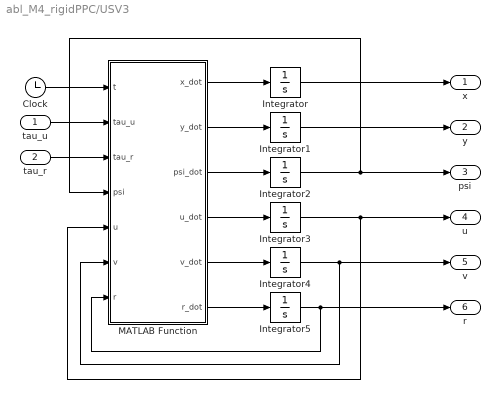
== system abl_M4_rigidPPC/USV3 ==
  tau_u : Inport
  tau_r : Inport  Port=2
  Clock : Clock
  Integrator : Integrator  InitialCondition=p_d_30(1)+8
  Integrator1 : Integrator  InitialCondition=p_d_30(2)+2
  Integrator{2..5} (4 alike) : Integrator
  MATLAB Function : MATLAB Function  TreatAsAtomicUnit=on
  x : Outport
  y : Outport  Port=2
  psi : Outport  Port=3
  u : Outport  Port=4
  v : Outport  Port=5
  r : Outport  Port=6
  wires:
  Integrator2/1 -> psi/1, MATLAB Function/4(psi)
  MATLAB Function/2(y_dot) -> Integrator1/1
  Integrator3/1 -> u/1, MATLAB Function/5(u)
  MATLAB Function/5(v_dot) -> Integrator4/1
  Integrator5/1 -> r/1, MATLAB Function/7(r)
  MATLAB Function/3(psi_dot) -> Integrator2/1
  MATLAB Function/6(r_dot) -> Integrator5/1
  tau_r/1 -> MATLAB Function/3(tau_r)
  Integrator4/1 -> v/1, MATLAB Function/6(v)
  Integrator/1 -> x/1
  MATLAB Function/4(u_dot) -> Integrator3/1
  MATLAB Function/1(x_dot) -> Integrator/1
  tau_u/1 -> MATLAB Function/2(tau_u)
  Integrator1/1 -> y/1
  Clock/1 -> MATLAB Function/1(t)

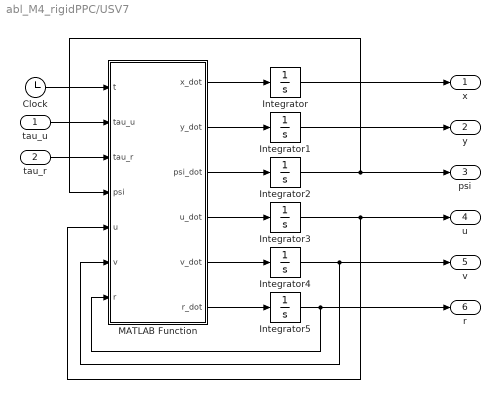
== system abl_M4_rigidPPC/USV7 ==
  tau_u : Inport
  tau_r : Inport  Port=2
  Clock : Clock
  Integrator : Integrator  InitialCondition=p_d_40(1)+8
  Integrator1 : Integrator  InitialCondition=p_d_40(2)+2
  Integrator{2..5} (4 alike) : Integrator
  MATLAB Function : MATLAB Function  TreatAsAtomicUnit=on
  x : Outport
  y : Outport  Port=2
  psi : Outport  Port=3
  u : Outport  Port=4
  v : Outport  Port=5
  r : Outport  Port=6
  wires:
  Integrator2/1 -> psi/1, MATLAB Function/4(psi)
  MATLAB Function/2(y_dot) -> Integrator1/1
  Integrator3/1 -> u/1, MATLAB Function/5(u)
  MATLAB Function/5(v_dot) -> Integrator4/1
  Integrator5/1 -> r/1, MATLAB Function/7(r)
  MATLAB Function/3(psi_dot) -> Integrator2/1
  MATLAB Function/6(r_dot) -> Integrator5/1
  tau_r/1 -> MATLAB Function/3(tau_r)
  Integrator4/1 -> v/1, MATLAB Function/6(v)
  Integrator/1 -> x/1
  MATLAB Function/4(u_dot) -> Integrator3/1
  MATLAB Function/1(x_dot) -> Integrator/1
  tau_u/1 -> MATLAB Function/2(tau_u)
  Integrator1/1 -> y/1
  Clock/1 -> MATLAB Function/1(t)

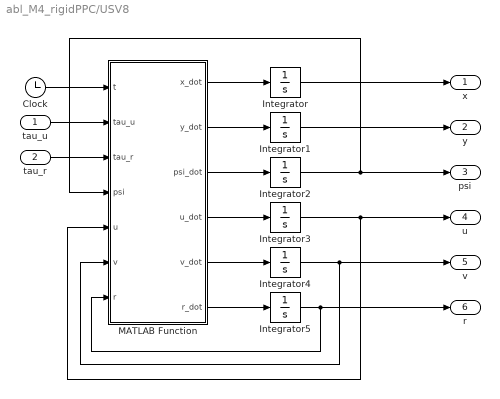
== system abl_M4_rigidPPC/USV8 ==
  tau_u : Inport
  tau_r : Inport  Port=2
  Clock : Clock
  Integrator : Integrator  InitialCondition=p_d_50(1)+8
  Integrator1 : Integrator  InitialCondition=p_d_50(2)+2
  Integrator{2..5} (4 alike) : Integrator
  MATLAB Function : MATLAB Function  TreatAsAtomicUnit=on
  x : Outport
  y : Outport  Port=2
  psi : Outport  Port=3
  u : Outport  Port=4
  v : Outport  Port=5
  r : Outport  Port=6
  wires:
  Integrator2/1 -> psi/1, MATLAB Function/4(psi)
  MATLAB Function/2(y_dot) -> Integrator1/1
  Integrator3/1 -> u/1, MATLAB Function/5(u)
  MATLAB Function/5(v_dot) -> Integrator4/1
  Integrator5/1 -> r/1, MATLAB Function/7(r)
  MATLAB Function/3(psi_dot) -> Integrator2/1
  MATLAB Function/6(r_dot) -> Integrator5/1
  tau_r/1 -> MATLAB Function/3(tau_r)
  Integrator4/1 -> v/1, MATLAB Function/6(v)
  Integrator/1 -> x/1
  MATLAB Function/4(u_dot) -> Integrator3/1
  MATLAB Function/1(x_dot) -> Integrator/1
  tau_u/1 -> MATLAB Function/2(tau_u)
  Integrator1/1 -> y/1
  Clock/1 -> MATLAB Function/1(t)

== system abl_M4_rigidPPC/USV9 ==
  tau_u : Inport
  tau_r : Inport  Port=2
  Clock : Clock
  Integrator : Integrator  InitialCondition=p_d_60(1)+8
  Integrator1 : Integrator  InitialCondition=p_d_60(2)+2
  Integrator{2..5} (4 alike) : Integrator
  MATLAB Function : MATLAB Function  TreatAsAtomicUnit=on
  x : Outport
  y : Outport  Port=2
  psi : Outport  Port=3
  u : Outport  Port=4
  v : Outport  Port=5
  r : Outport  Port=6
  wires:
  Integrator2/1 -> psi/1, MATLAB Function/4(psi)
  MATLAB Function/2(y_dot) -> Integrator1/1
  Integrator3/1 -> u/1, MATLAB Function/5(u)
  MATLAB Function/5(v_dot) -> Integrator4/1
  Integrator5/1 -> r/1, MATLAB Function/7(r)
  MATLAB Function/3(psi_dot) -> Integrator2/1
  MATLAB Function/6(r_dot) -> Integrator5/1
  tau_r/1 -> MATLAB Function/3(tau_r)
  Integrator4/1 -> v/1, MATLAB Function/6(v)
  Integrator/1 -> x/1
  MATLAB Function/4(u_dot) -> Integrator3/1
  MATLAB Function/1(x_dot) -> Integrator/1
  tau_u/1 -> MATLAB Function/2(tau_u)
  Integrator1/1 -> y/1
  Clock/1 -> MATLAB Function/1(t)

== system abl_M4_rigidPPC/Subsystem1/Subsystem ==
  t : Inport
  x : Inport  Port=2
  y : Inport  Port=3
  psi : Inport  Port=4
  "desire " : Inport  Port=5
  Guidence : MATLAB Function  TreatAsAtomicUnit=on
  Scope1 : Scope  NumInputPorts=2
  Scope5 : Scope  NumInputPorts=2
  psid : Outport
  psi_e : Outport  Port=2
  rhoe : Outport  Port=3
  wires:
  Guidence/2(psi_e) -> psi_e/1
  t/1 -> Guidence/1(t)
  psi/1 -> Guidence/5(psi)
  "desire "/1 -> Guidence/4(desire)
  Guidence/3(rhoe) -> rhoe/1
  x/1 -> Scope5/1, Guidence/2(x)
  y/1 -> Scope1/2, Guidence/3(y)
  Guidence/4(xd) -> Scope5/2
  Guidence/5(yd) -> Scope1/1
  Guidence/1(psid) -> psid/1

== system abl_M4_rigidPPC/Subsystem1/Subsystem1 ==
  psid : Inport
  Integrator{,1..3} (4 alike) : Integrator
  MATLAB Function1 : MATLAB Function  TreatAsAtomicUnit=on
  MATLAB Function2 : MATLAB Function  TreatAsAtomicUnit=on
  dpsid : Outport
  ddpsid : Outport  Port=2
  wires:
  MATLAB Function2/2(dotx2) -> Integrator1/1
  Integrator/1 -> MATLAB Function2/1(x1)
  MATLAB Function2/1(dotx1) -> Integrator/1
  psid/1 -> MATLAB Function2/3(psid)
  MATLAB Function1/2(dotx2) -> Integrator3/1
  MATLAB Function1/1(dotx1) -> Integrator2/1
  Integrator1/1 -> MATLAB Function1/3(psid), dpsid/1, MATLAB Function2/2(x2)
  Integrator2/1 -> MATLAB Function1/1(x1)
  Integrator3/1 -> ddpsid/1, MATLAB Function1/2(x2)

== system abl_M4_rigidPPC/Subsystem12/Subsystem ==
  t : Inport
  x : Inport  Port=2
  y : Inport  Port=3
  psi : Inport  Port=4
  "desire " : Inport  Port=5
  Guidence : MATLAB Function  TreatAsAtomicUnit=on
  Scope1 : Scope  NumInputPorts=2
  Scope5 : Scope  NumInputPorts=2
  psid : Outport
  psi_e : Outport  Port=2
  rhoe : Outport  Port=3
  wires:
  Guidence/2(psi_e) -> psi_e/1
  t/1 -> Guidence/1(t)
  psi/1 -> Guidence/5(psi)
  "desire "/1 -> Guidence/4(desire)
  Guidence/3(rhoe) -> rhoe/1
  x/1 -> Scope5/1, Guidence/2(x)
  y/1 -> Scope1/2, Guidence/3(y)
  Guidence/4(xd) -> Scope5/2
  Guidence/5(yd) -> Scope1/1
  Guidence/1(psid) -> psid/1

== system abl_M4_rigidPPC/Subsystem12/Subsystem1 ==
  psid : Inport
  Integrator{,1..3} (4 alike) : Integrator
  MATLAB Function1 : MATLAB Function  TreatAsAtomicUnit=on
  MATLAB Function2 : MATLAB Function  TreatAsAtomicUnit=on
  dpsid : Outport
  ddpsid : Outport  Port=2
  wires:
  MATLAB Function2/2(dotx2) -> Integrator1/1
  Integrator/1 -> MATLAB Function2/1(x1)
  MATLAB Function2/1(dotx1) -> Integrator/1
  psid/1 -> MATLAB Function2/3(psid)
  MATLAB Function1/2(dotx2) -> Integrator3/1
  MATLAB Function1/1(dotx1) -> Integrator2/1
  Integrator1/1 -> MATLAB Function1/3(psid), dpsid/1, MATLAB Function2/2(x2)
  Integrator2/1 -> MATLAB Function1/1(x1)
  Integrator3/1 -> ddpsid/1, MATLAB Function1/2(x2)

== system abl_M4_rigidPPC/Subsystem14/Subsystem ==
  t : Inport
  x : Inport  Port=2
  y : Inport  Port=3
  psi : Inport  Port=4
  "desire " : Inport  Port=5
  Guidence : MATLAB Function  TreatAsAtomicUnit=on
  Scope1 : Scope  NumInputPorts=2
  Scope5 : Scope  NumInputPorts=2
  psid : Outport
  psi_e : Outport  Port=2
  rhoe : Outport  Port=3
  wires:
  Guidence/2(psi_e) -> psi_e/1
  t/1 -> Guidence/1(t)
  psi/1 -> Guidence/5(psi)
  "desire "/1 -> Guidence/4(desire)
  Guidence/3(rhoe) -> rhoe/1
  x/1 -> Scope5/1, Guidence/2(x)
  y/1 -> Scope1/2, Guidence/3(y)
  Guidence/4(xd) -> Scope5/2
  Guidence/5(yd) -> Scope1/1
  Guidence/1(psid) -> psid/1

== system abl_M4_rigidPPC/Subsystem14/Subsystem1 ==
  psid : Inport
  Integrator{,1..3} (4 alike) : Integrator
  MATLAB Function1 : MATLAB Function  TreatAsAtomicUnit=on
  MATLAB Function2 : MATLAB Function  TreatAsAtomicUnit=on
  dpsid : Outport
  ddpsid : Outport  Port=2
  wires:
  MATLAB Function2/2(dotx2) -> Integrator1/1
  Integrator/1 -> MATLAB Function2/1(x1)
  MATLAB Function2/1(dotx1) -> Integrator/1
  psid/1 -> MATLAB Function2/3(psid)
  MATLAB Function1/2(dotx2) -> Integrator3/1
  MATLAB Function1/1(dotx1) -> Integrator2/1
  Integrator1/1 -> MATLAB Function1/3(psid), dpsid/1, MATLAB Function2/2(x2)
  Integrator2/1 -> MATLAB Function1/1(x1)
  Integrator3/1 -> ddpsid/1, MATLAB Function1/2(x2)

== system abl_M4_rigidPPC/Subsystem16/Subsystem ==
  t : Inport
  x : Inport  Port=2
  y : Inport  Port=3
  psi : Inport  Port=4
  "desire " : Inport  Port=5
  Guidence : MATLAB Function  TreatAsAtomicUnit=on
  Scope1 : Scope  NumInputPorts=2
  Scope5 : Scope  NumInputPorts=2
  psid : Outport
  psi_e : Outport  Port=2
  rhoe : Outport  Port=3
  wires:
  Guidence/2(psi_e) -> psi_e/1
  t/1 -> Guidence/1(t)
  psi/1 -> Guidence/5(psi)
  "desire "/1 -> Guidence/4(desire)
  Guidence/3(rhoe) -> rhoe/1
  x/1 -> Scope5/1, Guidence/2(x)
  y/1 -> Scope1/2, Guidence/3(y)
  Guidence/4(xd) -> Scope5/2
  Guidence/5(yd) -> Scope1/1
  Guidence/1(psid) -> psid/1

== system abl_M4_rigidPPC/Subsystem16/Subsystem1 ==
  psid : Inport
  Integrator{,1..3} (4 alike) : Integrator
  MATLAB Function1 : MATLAB Function  TreatAsAtomicUnit=on
  MATLAB Function2 : MATLAB Function  TreatAsAtomicUnit=on
  dpsid : Outport
  ddpsid : Outport  Port=2
  wires:
  MATLAB Function2/2(dotx2) -> Integrator1/1
  Integrator/1 -> MATLAB Function2/1(x1)
  MATLAB Function2/1(dotx1) -> Integrator/1
  psid/1 -> MATLAB Function2/3(psid)
  MATLAB Function1/2(dotx2) -> Integrator3/1
  MATLAB Function1/1(dotx1) -> Integrator2/1
  Integrator1/1 -> MATLAB Function1/3(psid), dpsid/1, MATLAB Function2/2(x2)
  Integrator2/1 -> MATLAB Function1/1(x1)
  Integrator3/1 -> ddpsid/1, MATLAB Function1/2(x2)

== system abl_M4_rigidPPC/Subsystem18/Subsystem ==
  t : Inport
  x : Inport  Port=2
  y : Inport  Port=3
  psi : Inport  Port=4
  "desire " : Inport  Port=5
  Guidence : MATLAB Function  TreatAsAtomicUnit=on
  Scope1 : Scope  NumInputPorts=2
  Scope5 : Scope  NumInputPorts=2
  psid : Outport
  psi_e : Outport  Port=2
  rhoe : Outport  Port=3
  wires:
  Guidence/2(psi_e) -> psi_e/1
  t/1 -> Guidence/1(t)
  psi/1 -> Guidence/5(psi)
  "desire "/1 -> Guidence/4(desire)
  Guidence/3(rhoe) -> rhoe/1
  x/1 -> Scope5/1, Guidence/2(x)
  y/1 -> Scope1/2, Guidence/3(y)
  Guidence/4(xd) -> Scope5/2
  Guidence/5(yd) -> Scope1/1
  Guidence/1(psid) -> psid/1

== system abl_M4_rigidPPC/Subsystem18/Subsystem1 ==
  psid : Inport
  Integrator{,1..3} (4 alike) : Integrator
  MATLAB Function1 : MATLAB Function  TreatAsAtomicUnit=on
  MATLAB Function2 : MATLAB Function  TreatAsAtomicUnit=on
  dpsid : Outport
  ddpsid : Outport  Port=2
  wires:
  MATLAB Function2/2(dotx2) -> Integrator1/1
  Integrator/1 -> MATLAB Function2/1(x1)
  MATLAB Function2/1(dotx1) -> Integrator/1
  psid/1 -> MATLAB Function2/3(psid)
  MATLAB Function1/2(dotx2) -> Integrator3/1
  MATLAB Function1/1(dotx1) -> Integrator2/1
  Integrator1/1 -> MATLAB Function1/3(psid), dpsid/1, MATLAB Function2/2(x2)
  Integrator2/1 -> MATLAB Function1/1(x1)
  Integrator3/1 -> ddpsid/1, MATLAB Function1/2(x2)

== system abl_M4_rigidPPC/Subsystem3/Subsystem ==
  t : Inport
  x : Inport  Port=2
  y : Inport  Port=3
  psi : Inport  Port=4
  "desire " : Inport  Port=5
  Guidence : MATLAB Function  TreatAsAtomicUnit=on
  Scope1 : Scope  NumInputPorts=2
  Scope5 : Scope  NumInputPorts=2
  psid : Outport
  psi_e : Outport  Port=2
  rhoe : Outport  Port=3
  wires:
  Guidence/2(psi_e) -> psi_e/1
  t/1 -> Guidence/1(t)
  psi/1 -> Guidence/5(psi)
  "desire "/1 -> Guidence/4(desire)
  Guidence/3(rhoe) -> rhoe/1
  x/1 -> Scope5/1, Guidence/2(x)
  y/1 -> Scope1/2, Guidence/3(y)
  Guidence/4(xd) -> Scope5/2
  Guidence/5(yd) -> Scope1/1
  Guidence/1(psid) -> psid/1

== system abl_M4_rigidPPC/Subsystem3/Subsystem1 ==
  psid : Inport
  Integrator{,1..3} (4 alike) : Integrator
  MATLAB Function1 : MATLAB Function  TreatAsAtomicUnit=on
  MATLAB Function2 : MATLAB Function  TreatAsAtomicUnit=on
  dpsid : Outport
  ddpsid : Outport  Port=2
  wires:
  MATLAB Function2/2(dotx2) -> Integrator1/1
  Integrator/1 -> MATLAB Function2/1(x1)
  MATLAB Function2/1(dotx1) -> Integrator/1
  psid/1 -> MATLAB Function2/3(psid)
  MATLAB Function1/2(dotx2) -> Integrator3/1
  MATLAB Function1/1(dotx1) -> Integrator2/1
  Integrator1/1 -> MATLAB Function1/3(psid), dpsid/1, MATLAB Function2/2(x2)
  Integrator2/1 -> MATLAB Function1/1(x1)
  Integrator3/1 -> ddpsid/1, MATLAB Function1/2(x2)

== matlab function abl_M4_rigidPPC/MATLAB Function2 ==
  settings: updateMethod=DISCRETE
  data: t input; p0 input; v0 input; dp0 output; dv0 output
function [dp0, dv0] = Leader_Model(t,p0, v0)
    % 领航者（移动目标）动力学模型
    % 输入: 
    %   p0: 领航者当前位置 (例如 2x1 向量)
    %   v0: 领航者当前速度 (例如 2x1 向量)
    %   u0: 领航者加速度控制输入 (可在外部接Sine Wave或常数)
    % 输出: 位置和速度的导数
    
    dp0 = v0; 
    dv0 = [0.08*sin(0.05*t);0.08*cos(0.05*t)]; 
end
